simulink model "Roll_Autopilot"  (R2017b)
settings: Solver=VariableStepAuto  StartTime=0.0  StopTime=10.0  RelTol=1e-3
model workspace (MAT data in the model file):
  MCOS : class17 (value not decoded)
undefined symbols (not defined in the file): contractAfterSimulation, contractBeforeSimulation, ContractBlock, ContractEnsureBlock, ContractGuaranteeBlock, ContractModeBlock, ContractRequireBlock, ContractValidatorBlock, saveValidatorParameters, Ts
libraries: cocosimLibs x20, simulink x2
(part 2 of 2)

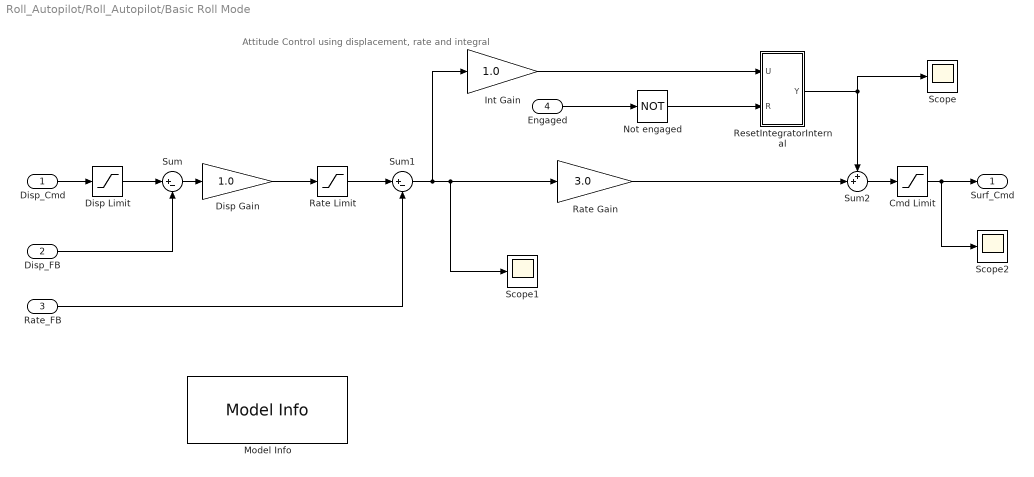
== system Roll_Autopilot/Roll_Autopilot/Basic Roll Mode ==
  note: Attitude Control using displacement, rate and integral
  Disp_Cmd : Inport  OutDataTypeStr=double  PortDimensions=1
  "Disp_FB " : Inport  Port=2  OutDataTypeStr=double  PortDimensions=1  SampleTime=1/40
  Rate_FB : Inport  Port=3  OutDataTypeStr=double  PortDimensions=1  SampleTime=1/40
  Engaged : Inport  Port=4  OutDataTypeStr=boolean  PortDimensions=1  SampleTime=1/40
  Cmd Limit : Saturate  UpperLimit=15  LowerLimit=-15
      settings: AttributesFormatString=%<LowerLimit> to %<UpperLimit> (deg)
  Disp Gain : Gain  Gain=1.0
  Disp Limit : Saturate  UpperLimit=30  LowerLimit=-30
      settings: AttributesFormatString=%<LowerLimit> to %<UpperLimit> (deg)
  Int Gain : Gain  Gain=1.0
  Model Info : simulink/Model-Wide Utilities/Model Info  Frame=on  DisplayStringWithTags=|  HorizontalTextAlignment=Left  LeftAlignmentValue=0.02
      | Attitude Controller
      | Author: %<LastModifiedBy>
      | Version: %<ModelVersion>
      | Date: %<LastModificationDate>
  Not engaged : Logic  Operator=NOT  IconShape=distinctive  AllPortsSameDT=off  OutDataTypeStr=boolean
  Rate Gain : Gain  Gain=3.0
  Rate Limit : Saturate  UpperLimit=6  LowerLimit=-6
      settings: AttributesFormatString=%<LowerLimit> to %<UpperLimit> (deg/sec)
  ResetIntegratorInternal : Subsystem
  Scope : Scope
  Scope1 : Scope
  Scope2 : Scope
  Sum : Sum  Inputs=|+-
  Sum1 : Sum  Inputs=|+-
  Sum2 : Sum  Inputs=++|
  Surf_Cmd : Outport  OutDataTypeStr=double  PortDimensions=1  SampleTime=1/40  VectorParamsAs1DForOutWhenUnconnected=off
  wires:
  Engaged/1 -> Not engaged/1
  Disp_Cmd/1 -> Disp Limit/1
  Rate Limit/1 -> Sum1/1
  ResetIntegratorInternal/1(Y) -> Sum2/1, Scope/1
  Not engaged/1 -> ResetIntegratorInternal/2(R)
  Rate_FB/1 -> Sum1/2
  Sum1/1 -> Int Gain/1, Scope1/1, Rate Gain/1
  Cmd Limit/1 -> Scope2/1, Surf_Cmd/1
  Rate Gain/1 -> Sum2/2
  Disp Gain/1 -> Rate Limit/1
  Sum/1 -> Disp Gain/1
  "Disp_FB "/1 -> Sum/2
  Disp Limit/1 -> Sum/1
  Sum2/1 -> Cmd Limit/1
  Int Gain/1 -> ResetIntegratorInternal/1(U)

== system Roll_Autopilot/Roll_Autopilot/Heading Mode ==
  Psi Ref : Inport  OutDataTypeStr=double  PortDimensions=1  SampleTime=1/40  Interpolate=off
  Psi : Inport  Port=2  OutDataTypeStr=double  PortDimensions=1  SampleTime=1/40  Interpolate=off
  TAS : Inport  Port=3  OutDataTypeStr=double  PortDimensions=1  SampleTime=1/40  Interpolate=off
  Disp Gain : Gain  Gain=0.015
  Model Info : simulink/Model-Wide Utilities/Model Info  Frame=on  DisplayStringWithTags=|  HorizontalTextAlignment=Left  LeftAlignmentValue=0.02
      | Heading Mode
      | Author: %<LastModifiedBy>
      | Version: %<ModelVersion>
      | Date: %<LastModificationDate>
  Product : Product  RndMeth=Zero
  angle diff : Subsystem
  Phi Cmd : Outport  OutDataTypeStr=double  PortDimensions=1  SampleTime=1/40  VectorParamsAs1DForOutWhenUnconnected=off
  wires:
  Psi Ref/1 -> angle diff/1(plus)
  angle diff/1(diff) -> Disp Gain/1  "hdgError"
  TAS/1 -> Product/2
  Disp Gain/1 -> Product/1
  Psi/1 -> angle diff/2(minus)
  Product/1 -> Phi Cmd/1

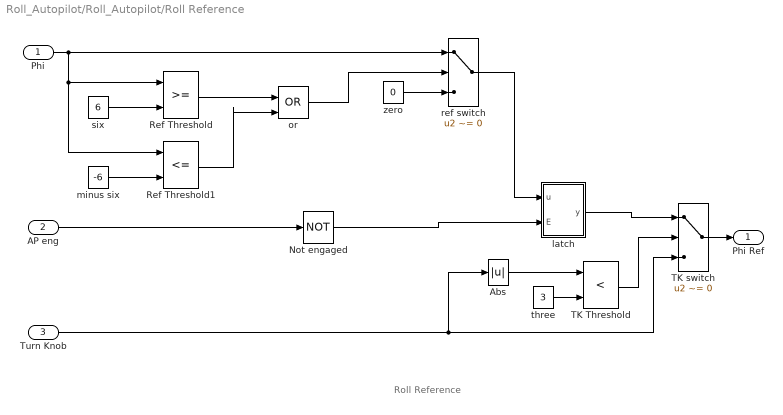
== system Roll_Autopilot/Roll_Autopilot/Roll Reference ==
  note: Roll Reference
  Phi : Inport
  AP eng : Inport  Port=2
  Turn Knob : Inport  Port=3
  Abs : Abs
  Not engaged : Logic  Operator=NOT  IconShape=distinctive  AllPortsSameDT=off  OutDataTypeStr=boolean
  Ref Threshold : RelationalOperator  OutDataTypeStr=boolean  RndMeth=Nearest  InputSameDT=on
  Ref Threshold1 : RelationalOperator  Operator=<=  OutDataTypeStr=boolean  RndMeth=Nearest  InputSameDT=on
  TK Threshold : RelationalOperator  Operator=<  OutDataTypeStr=boolean  RndMeth=Nearest  InputSameDT=on
  TK switch : Switch  Criteria=u2 ~= 0
  latch : Subsystem
  minus six : Constant  Value=-6
  or : Logic  Operator=OR  IconShape=distinctive  OutDataTypeStr=boolean
  ref switch : Switch  Criteria=u2 ~= 0
  six : Constant  Value=6
  three : Constant  Value=3  OutDataTypeStr=double
  zero : Constant  Value=0
  Phi Ref : Outport  VectorParamsAs1DForOutWhenUnconnected=off
  wires:
  minus six/1 -> Ref Threshold1/2
  Ref Threshold1/1 -> or/2
  Ref Threshold/1 -> or/1
  or/1 -> ref switch/2
  zero/1 -> ref switch/3
  six/1 -> Ref Threshold/2
  TK switch/1 -> Phi Ref/1
  AP eng/1 -> Not engaged/1
  Phi/1 -> Ref Threshold1/1, Ref Threshold/1, ref switch/1
  Abs/1 -> TK Threshold/1
  three/1 -> TK Threshold/2
  Turn Knob/1 -> Abs/1, TK switch/3
  TK Threshold/1 -> TK switch/2
  latch/1(y) -> TK switch/1
  ref switch/1 -> latch/1(u)
  Not engaged/1 -> latch/2(E)

== system Roll_Autopilot/Roll_Autopilot_RollAutopilotSpec1/AP-001 ==
  In1 : Inport
  guarantee : Outport  OutDataTypeStr=boolean
  wires:
  In1/1 -> guarantee/1

== system Roll_Autopilot/Roll_Autopilot_RollAutopilotSpec1/AP-003A ==
  In1 : Inport
  guarantee : Outport  OutDataTypeStr=boolean
  wires:
  In1/1 -> guarantee/1

== system Roll_Autopilot/Roll_Autopilot_RollAutopilotSpec1/AP-003B ==
  In1 : Inport
  guarantee : Outport  OutDataTypeStr=boolean
  wires:
  In1/1 -> guarantee/1

== system Roll_Autopilot/Roll_Autopilot_RollAutopilotSpec1/AP-003C ==
  In1 : Inport
  guarantee : Outport  OutDataTypeStr=boolean
  wires:
  In1/1 -> guarantee/1

== system Roll_Autopilot/Roll_Autopilot_RollAutopilotSpec1/AP-003D ==
  In1 : Inport
  guarantee : Outport  OutDataTypeStr=boolean
  wires:
  In1/1 -> guarantee/1

== system Roll_Autopilot/Roll_Autopilot_RollAutopilotSpec1/AP-007 ==
  In1 : Inport
  guarantee : Outport  OutDataTypeStr=boolean
  wires:
  In1/1 -> guarantee/1

== system Roll_Autopilot/Roll_Autopilot_RollAutopilotSpec1/H_call ==
  H_X : Inport  OutDataTypeStr=boolean
  Arrow_xxH_1_ni_23 : Delay  DelayLength=1  InitialCondition=1
  PRE_xxH_2 : Delay  DelayLength=1  InitialCondition=0
  branch_6_IF : Switch  Criteria=u2 ~= 0
  xxH_1_ni_23_init : Constant  Value=0  OutDataTypeStr=boolean
  xxH_3_operator : Logic  AllPortsSameDT=off  OutDataTypeStr=boolean
  H_Y : Outport
  wires:
  PRE_xxH_2/1 -> xxH_3_operator/2
  xxH_3_operator/1 -> branch_6_IF/3
  Arrow_xxH_1_ni_23/1 -> branch_6_IF/2
  xxH_1_ni_23_init/1 -> Arrow_xxH_1_ni_23/1
  branch_6_IF/1 -> H_Y/1, PRE_xxH_2/1
  H_X/1 -> xxH_3_operator/1, branch_6_IF/1

== system Roll_Autopilot/Roll_Autopilot_RollAutopilotSpec1/H_call1 ==
  H_X : Inport  OutDataTypeStr=boolean
  Arrow_xxH_1_ni_23 : Delay  DelayLength=1  InitialCondition=1
  PRE_xxH_2 : Delay  DelayLength=1  InitialCondition=0
  branch_6_IF : Switch  Criteria=u2 ~= 0
  xxH_1_ni_23_init : Constant  Value=0  OutDataTypeStr=boolean
  xxH_3_operator : Logic  AllPortsSameDT=off  OutDataTypeStr=boolean
  H_Y : Outport
  wires:
  PRE_xxH_2/1 -> xxH_3_operator/2
  xxH_3_operator/1 -> branch_6_IF/3
  Arrow_xxH_1_ni_23/1 -> branch_6_IF/2
  xxH_1_ni_23_init/1 -> Arrow_xxH_1_ni_23/1
  branch_6_IF/1 -> H_Y/1, PRE_xxH_2/1
  H_X/1 -> xxH_3_operator/1, branch_6_IF/1

== system Roll_Autopilot/Roll_Autopilot_RollAutopilotSpec1/H_call11 ==
  H_X : Inport  OutDataTypeStr=boolean
  Arrow_xxH_1_ni_23 : Delay  DelayLength=1  InitialCondition=1
  PRE_xxH_2 : Delay  DelayLength=1  InitialCondition=0
  branch_6_IF : Switch  Criteria=u2 ~= 0
  xxH_1_ni_23_init : Constant  Value=0  OutDataTypeStr=boolean
  xxH_3_operator : Logic  AllPortsSameDT=off  OutDataTypeStr=boolean
  H_Y : Outport
  wires:
  PRE_xxH_2/1 -> xxH_3_operator/2
  xxH_3_operator/1 -> branch_6_IF/3
  Arrow_xxH_1_ni_23/1 -> branch_6_IF/2
  xxH_1_ni_23_init/1 -> Arrow_xxH_1_ni_23/1
  branch_6_IF/1 -> H_Y/1, PRE_xxH_2/1
  H_X/1 -> xxH_3_operator/1, branch_6_IF/1

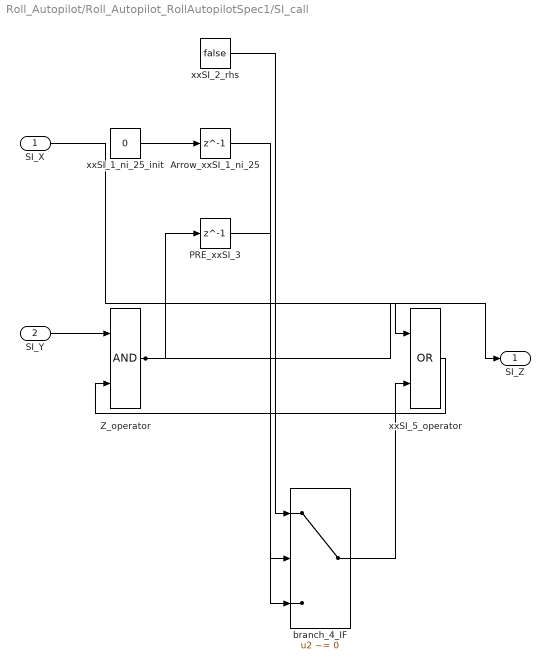
== system Roll_Autopilot/Roll_Autopilot_RollAutopilotSpec1/SI_call ==
  SI_X : Inport  OutDataTypeStr=boolean
  SI_Y : Inport  Port=2  OutDataTypeStr=boolean
  Arrow_xxSI_1_ni_25 : Delay  DelayLength=1  InitialCondition=1
  PRE_xxSI_3 : Delay  DelayLength=1  InitialCondition=0
  Z_operator : Logic  AllPortsSameDT=off  OutDataTypeStr=boolean
  branch_4_IF : Switch  Criteria=u2 ~= 0
  xxSI_1_ni_25_init : Constant  Value=0  OutDataTypeStr=boolean
  xxSI_2_rhs : Constant  Value=false  OutDataTypeStr=boolean
  xxSI_5_operator : Logic  Operator=OR  AllPortsSameDT=off  OutDataTypeStr=boolean
  SI_Z : Outport
  wires:
  branch_4_IF/1 -> xxSI_5_operator/2
  SI_X/1 -> xxSI_5_operator/1
  PRE_xxSI_3/1 -> branch_4_IF/3
  Arrow_xxSI_1_ni_25/1 -> branch_4_IF/2
  xxSI_2_rhs/1 -> branch_4_IF/1
  xxSI_5_operator/1 -> Z_operator/2
  SI_Y/1 -> Z_operator/1
  xxSI_1_ni_25_init/1 -> Arrow_xxSI_1_ni_25/1
  Z_operator/1 -> SI_Z/1, PRE_xxSI_3/1

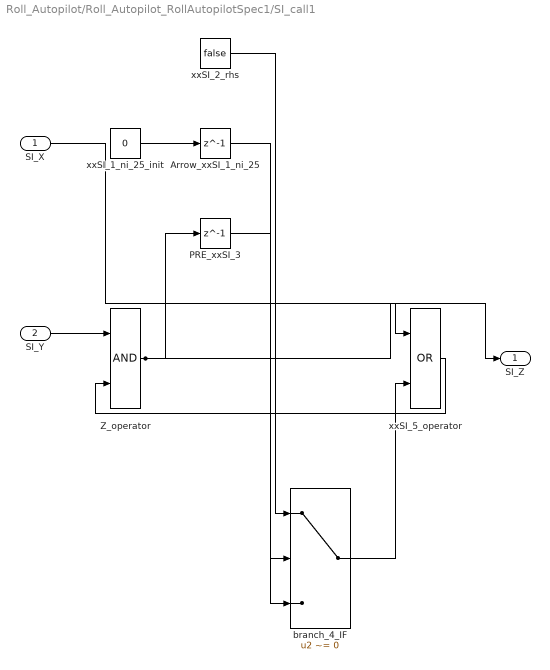
== system Roll_Autopilot/Roll_Autopilot_RollAutopilotSpec1/SI_call1 ==
  SI_X : Inport  OutDataTypeStr=boolean
  SI_Y : Inport  Port=2  OutDataTypeStr=boolean
  Arrow_xxSI_1_ni_25 : Delay  DelayLength=1  InitialCondition=1
  PRE_xxSI_3 : Delay  DelayLength=1  InitialCondition=0
  Z_operator : Logic  AllPortsSameDT=off  OutDataTypeStr=boolean
  branch_4_IF : Switch  Criteria=u2 ~= 0
  xxSI_1_ni_25_init : Constant  Value=0  OutDataTypeStr=boolean
  xxSI_2_rhs : Constant  Value=false  OutDataTypeStr=boolean
  xxSI_5_operator : Logic  Operator=OR  AllPortsSameDT=off  OutDataTypeStr=boolean
  SI_Z : Outport
  wires:
  branch_4_IF/1 -> xxSI_5_operator/2
  SI_X/1 -> xxSI_5_operator/1
  PRE_xxSI_3/1 -> branch_4_IF/3
  Arrow_xxSI_1_ni_25/1 -> branch_4_IF/2
  xxSI_2_rhs/1 -> branch_4_IF/1
  xxSI_5_operator/1 -> Z_operator/2
  SI_Y/1 -> Z_operator/1
  xxSI_1_ni_25_init/1 -> Arrow_xxSI_1_ni_25/1
  Z_operator/1 -> SI_Z/1, PRE_xxSI_3/1

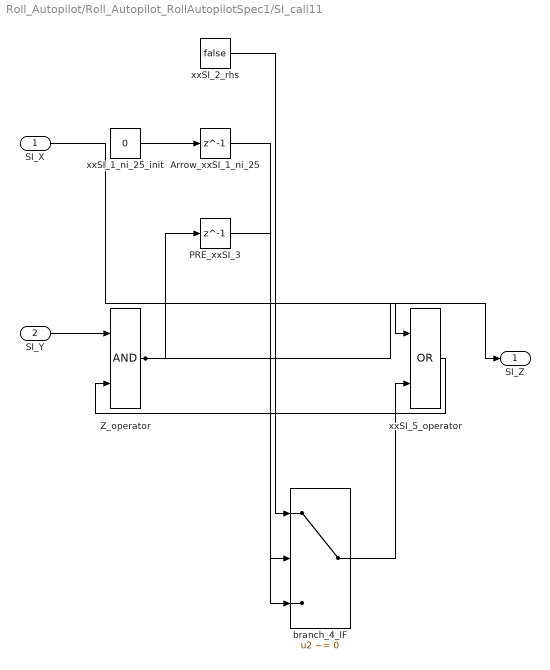
== system Roll_Autopilot/Roll_Autopilot_RollAutopilotSpec1/SI_call11 ==
  SI_X : Inport  OutDataTypeStr=boolean
  SI_Y : Inport  Port=2  OutDataTypeStr=boolean
  Arrow_xxSI_1_ni_25 : Delay  DelayLength=1  InitialCondition=1
  PRE_xxSI_3 : Delay  DelayLength=1  InitialCondition=0
  Z_operator : Logic  AllPortsSameDT=off  OutDataTypeStr=boolean
  branch_4_IF : Switch  Criteria=u2 ~= 0
  xxSI_1_ni_25_init : Constant  Value=0  OutDataTypeStr=boolean
  xxSI_2_rhs : Constant  Value=false  OutDataTypeStr=boolean
  xxSI_5_operator : Logic  Operator=OR  AllPortsSameDT=off  OutDataTypeStr=boolean
  SI_Z : Outport
  wires:
  branch_4_IF/1 -> xxSI_5_operator/2
  SI_X/1 -> xxSI_5_operator/1
  PRE_xxSI_3/1 -> branch_4_IF/3
  Arrow_xxSI_1_ni_25/1 -> branch_4_IF/2
  xxSI_2_rhs/1 -> branch_4_IF/1
  xxSI_5_operator/1 -> Z_operator/2
  SI_Y/1 -> Z_operator/1
  xxSI_1_ni_25_init/1 -> Arrow_xxSI_1_ni_25/1
  Z_operator/1 -> SI_Z/1, PRE_xxSI_3/1

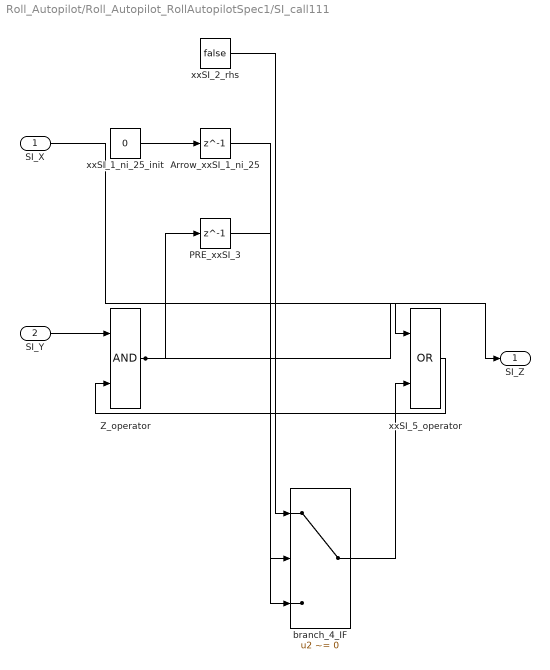
== system Roll_Autopilot/Roll_Autopilot_RollAutopilotSpec1/SI_call111 ==
  SI_X : Inport  OutDataTypeStr=boolean
  SI_Y : Inport  Port=2  OutDataTypeStr=boolean
  Arrow_xxSI_1_ni_25 : Delay  DelayLength=1  InitialCondition=1
  PRE_xxSI_3 : Delay  DelayLength=1  InitialCondition=0
  Z_operator : Logic  AllPortsSameDT=off  OutDataTypeStr=boolean
  branch_4_IF : Switch  Criteria=u2 ~= 0
  xxSI_1_ni_25_init : Constant  Value=0  OutDataTypeStr=boolean
  xxSI_2_rhs : Constant  Value=false  OutDataTypeStr=boolean
  xxSI_5_operator : Logic  Operator=OR  AllPortsSameDT=off  OutDataTypeStr=boolean
  SI_Z : Outport
  wires:
  branch_4_IF/1 -> xxSI_5_operator/2
  SI_X/1 -> xxSI_5_operator/1
  PRE_xxSI_3/1 -> branch_4_IF/3
  Arrow_xxSI_1_ni_25/1 -> branch_4_IF/2
  xxSI_2_rhs/1 -> branch_4_IF/1
  xxSI_5_operator/1 -> Z_operator/2
  SI_Y/1 -> Z_operator/1
  xxSI_1_ni_25_init/1 -> Arrow_xxSI_1_ni_25/1
  Z_operator/1 -> SI_Z/1, PRE_xxSI_3/1

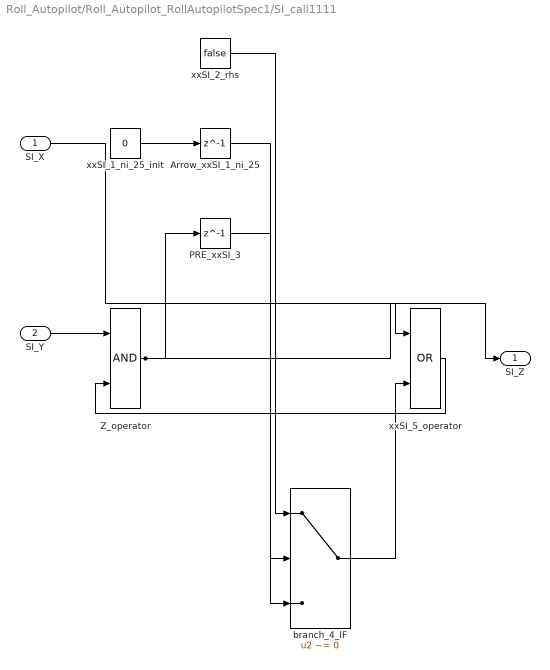
== system Roll_Autopilot/Roll_Autopilot_RollAutopilotSpec1/SI_call1111 ==
  SI_X : Inport  OutDataTypeStr=boolean
  SI_Y : Inport  Port=2  OutDataTypeStr=boolean
  Arrow_xxSI_1_ni_25 : Delay  DelayLength=1  InitialCondition=1
  PRE_xxSI_3 : Delay  DelayLength=1  InitialCondition=0
  Z_operator : Logic  AllPortsSameDT=off  OutDataTypeStr=boolean
  branch_4_IF : Switch  Criteria=u2 ~= 0
  xxSI_1_ni_25_init : Constant  Value=0  OutDataTypeStr=boolean
  xxSI_2_rhs : Constant  Value=false  OutDataTypeStr=boolean
  xxSI_5_operator : Logic  Operator=OR  AllPortsSameDT=off  OutDataTypeStr=boolean
  SI_Z : Outport
  wires:
  branch_4_IF/1 -> xxSI_5_operator/2
  SI_X/1 -> xxSI_5_operator/1
  PRE_xxSI_3/1 -> branch_4_IF/3
  Arrow_xxSI_1_ni_25/1 -> branch_4_IF/2
  xxSI_2_rhs/1 -> branch_4_IF/1
  xxSI_5_operator/1 -> Z_operator/2
  SI_Y/1 -> Z_operator/1
  xxSI_1_ni_25_init/1 -> Arrow_xxSI_1_ni_25/1
  Z_operator/1 -> SI_Z/1, PRE_xxSI_3/1

== system Roll_Autopilot/Roll_Autopilot_RollAutopilotSpec1/SI_call11111 ==
  SI_X : Inport  OutDataTypeStr=boolean
  SI_Y : Inport  Port=2  OutDataTypeStr=boolean
  Arrow_xxSI_1_ni_25 : Delay  DelayLength=1  InitialCondition=1
  PRE_xxSI_3 : Delay  DelayLength=1  InitialCondition=0
  Z_operator : Logic  AllPortsSameDT=off  OutDataTypeStr=boolean
  branch_4_IF : Switch  Criteria=u2 ~= 0
  xxSI_1_ni_25_init : Constant  Value=0  OutDataTypeStr=boolean
  xxSI_2_rhs : Constant  Value=false  OutDataTypeStr=boolean
  xxSI_5_operator : Logic  Operator=OR  AllPortsSameDT=off  OutDataTypeStr=boolean
  SI_Z : Outport
  wires:
  branch_4_IF/1 -> xxSI_5_operator/2
  SI_X/1 -> xxSI_5_operator/1
  PRE_xxSI_3/1 -> branch_4_IF/3
  Arrow_xxSI_1_ni_25/1 -> branch_4_IF/2
  xxSI_2_rhs/1 -> branch_4_IF/1
  xxSI_5_operator/1 -> Z_operator/2
  SI_Y/1 -> Z_operator/1
  xxSI_1_ni_25_init/1 -> Arrow_xxSI_1_ni_25/1
  Z_operator/1 -> SI_Z/1, PRE_xxSI_3/1

== system Roll_Autopilot/Roll_Autopilot_RollAutopilotSpec1/SI_call111111 ==
  SI_X : Inport  OutDataTypeStr=boolean
  SI_Y : Inport  Port=2  OutDataTypeStr=boolean
  Arrow_xxSI_1_ni_25 : Delay  DelayLength=1  InitialCondition=1
  PRE_xxSI_3 : Delay  DelayLength=1  InitialCondition=0
  Z_operator : Logic  AllPortsSameDT=off  OutDataTypeStr=boolean
  branch_4_IF : Switch  Criteria=u2 ~= 0
  xxSI_1_ni_25_init : Constant  Value=0  OutDataTypeStr=boolean
  xxSI_2_rhs : Constant  Value=false  OutDataTypeStr=boolean
  xxSI_5_operator : Logic  Operator=OR  AllPortsSameDT=off  OutDataTypeStr=boolean
  SI_Z : Outport
  wires:
  branch_4_IF/1 -> xxSI_5_operator/2
  SI_X/1 -> xxSI_5_operator/1
  PRE_xxSI_3/1 -> branch_4_IF/3
  Arrow_xxSI_1_ni_25/1 -> branch_4_IF/2
  xxSI_2_rhs/1 -> branch_4_IF/1
  xxSI_5_operator/1 -> Z_operator/2
  SI_Y/1 -> Z_operator/1
  xxSI_1_ni_25_init/1 -> Arrow_xxSI_1_ni_25/1
  Z_operator/1 -> SI_Z/1, PRE_xxSI_3/1

== system Roll_Autopilot/Roll_Autopilot_RollAutopilotSpec1/SI_call1111111 ==
  SI_X : Inport  OutDataTypeStr=boolean
  SI_Y : Inport  Port=2  OutDataTypeStr=boolean
  Arrow_xxSI_1_ni_25 : Delay  DelayLength=1  InitialCondition=1
  PRE_xxSI_3 : Delay  DelayLength=1  InitialCondition=0
  Z_operator : Logic  AllPortsSameDT=off  OutDataTypeStr=boolean
  branch_4_IF : Switch  Criteria=u2 ~= 0
  xxSI_1_ni_25_init : Constant  Value=0  OutDataTypeStr=boolean
  xxSI_2_rhs : Constant  Value=false  OutDataTypeStr=boolean
  xxSI_5_operator : Logic  Operator=OR  AllPortsSameDT=off  OutDataTypeStr=boolean
  SI_Z : Outport
  wires:
  branch_4_IF/1 -> xxSI_5_operator/2
  SI_X/1 -> xxSI_5_operator/1
  PRE_xxSI_3/1 -> branch_4_IF/3
  Arrow_xxSI_1_ni_25/1 -> branch_4_IF/2
  xxSI_2_rhs/1 -> branch_4_IF/1
  xxSI_5_operator/1 -> Z_operator/2
  SI_Y/1 -> Z_operator/1
  xxSI_1_ni_25_init/1 -> Arrow_xxSI_1_ni_25/1
  Z_operator/1 -> SI_Z/1, PRE_xxSI_3/1

== system Roll_Autopilot/Roll_Autopilot_RollAutopilotSpec1/SI_call11111111 ==
  SI_X : Inport  OutDataTypeStr=boolean
  SI_Y : Inport  Port=2  OutDataTypeStr=boolean
  Arrow_xxSI_1_ni_25 : Delay  DelayLength=1  InitialCondition=1
  PRE_xxSI_3 : Delay  DelayLength=1  InitialCondition=0
  Z_operator : Logic  AllPortsSameDT=off  OutDataTypeStr=boolean
  branch_4_IF : Switch  Criteria=u2 ~= 0
  xxSI_1_ni_25_init : Constant  Value=0  OutDataTypeStr=boolean
  xxSI_2_rhs : Constant  Value=false  OutDataTypeStr=boolean
  xxSI_5_operator : Logic  Operator=OR  AllPortsSameDT=off  OutDataTypeStr=boolean
  SI_Z : Outport
  wires:
  branch_4_IF/1 -> xxSI_5_operator/2
  SI_X/1 -> xxSI_5_operator/1
  PRE_xxSI_3/1 -> branch_4_IF/3
  Arrow_xxSI_1_ni_25/1 -> branch_4_IF/2
  xxSI_2_rhs/1 -> branch_4_IF/1
  xxSI_5_operator/1 -> Z_operator/2
  SI_Y/1 -> Z_operator/1
  xxSI_1_ni_25_init/1 -> Arrow_xxSI_1_ni_25/1
  Z_operator/1 -> SI_Z/1, PRE_xxSI_3/1

== system Roll_Autopilot/Roll_Autopilot_RollAutopilotSpec1/hdg_hold_mode ==
  note: Shouldn't not be edited
  require : Inport  OutDataTypeStr=boolean
  ensure : Inport  Port=2  OutDataTypeStr=boolean
  and : Logic  Operator=NOT  IconShape=distinctive  AllPortsSameDT=off  OutDataTypeStr=boolean
  or : Logic  Operator=OR  IconShape=distinctive  AllPortsSameDT=off  OutDataTypeStr=boolean
  mode : Outport
  wires:
  or/1 -> mode/1
  ensure/1 -> or/2
  and/1 -> or/1
  require/1 -> and/1

== system Roll_Autopilot/Roll_Autopilot_RollAutopilotSpec1/hdg_hold_mode_ensure ==
  In1 : Inport
  ensure : Outport  OutDataTypeStr=boolean
  wires:
  In1/1 -> ensure/1

== system Roll_Autopilot/Roll_Autopilot_RollAutopilotSpec1/hdg_hold_mode_require ==
  In1 : Inport
  require : Outport  OutDataTypeStr=boolean
  wires:
  In1/1 -> require/1

== system Roll_Autopilot/Roll_Autopilot_RollAutopilotSpec1/roll_hold_mode ==
  note: Shouldn't not be edited
  require : Inport  OutDataTypeStr=boolean
  ensure : Inport  Port=2  OutDataTypeStr=boolean
  and : Logic  Operator=NOT  IconShape=distinctive  AllPortsSameDT=off  OutDataTypeStr=boolean
  or : Logic  Operator=OR  IconShape=distinctive  AllPortsSameDT=off  OutDataTypeStr=boolean
  mode : Outport
  wires:
  or/1 -> mode/1
  ensure/1 -> or/2
  and/1 -> or/1
  require/1 -> and/1

== system Roll_Autopilot/Roll_Autopilot_RollAutopilotSpec1/roll_hold_mode_ensure ==
  In1 : Inport
  ensure : Outport  OutDataTypeStr=boolean
  wires:
  In1/1 -> ensure/1

== system Roll_Autopilot/Roll_Autopilot_RollAutopilotSpec1/roll_hold_mode_require ==
  In1 : Inport
  require : Outport  OutDataTypeStr=boolean
  wires:
  In1/1 -> require/1

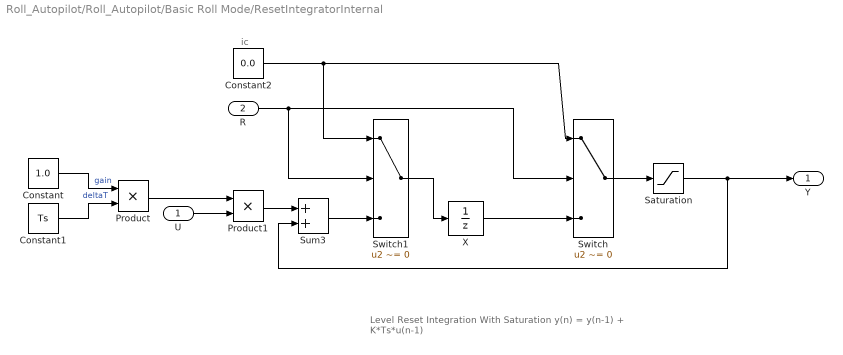
== system Roll_Autopilot/Roll_Autopilot/Basic Roll Mode/ResetIntegratorInternal ==
  note: ic
  note: Level Reset Integration With Saturation
      | y(n) = y(n-1) + K*Ts*u(n-1)
  U : Inport
  R : Inport  Port=2
  Constant : Constant  Value=1.0
  Constant1 : Constant  Value=Ts
  Constant2 : Constant  Value=0.0
  Product : Product  RndMeth=Zero
  Product1 : Product  RndMeth=Zero
  Saturation : Saturate  UpperLimit=5  LowerLimit=-5
  Sum3 : Sum
  Switch : Switch  Criteria=u2 ~= 0
  Switch1 : Switch  Criteria=u2 ~= 0
  X : UnitDelay  SampleTime=Ts  HasFrameUpgradeWarning=on
  Y : Outport  VectorParamsAs1DForOutWhenUnconnected=off
  wires:
  Product1/1 -> Sum3/1
  U/1 -> Product1/2
  Sum3/1 -> Switch1/3
  Product/1 -> Product1/1
  Switch/1 -> Saturation/1
  Constant2/1 -> Switch1/1, Switch/1
  Constant1/1 -> Product/2  "deltaT"
  Switch1/1 -> X/1
  Constant/1 -> Product/1  "gain"
  Saturation/1 -> Y/1, Sum3/2
  R/1 -> Switch1/2, Switch/2
  X/1 -> Switch/3

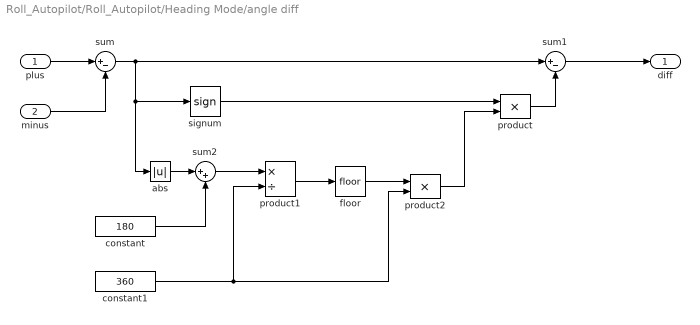
== system Roll_Autopilot/Roll_Autopilot/Heading Mode/angle diff ==
  plus : Inport  OutDataTypeStr=double
  minus : Inport  Port=2  OutDataTypeStr=double
  abs : Abs  ZeroCross=off
  constant : Constant  Value=180
  constant1 : Constant  Value=360
  floor : Rounding
  product : Product  RndMeth=Zero  InputSameDT=on  OutDataTypeStr=Inherit: Same as first input
  product1 : Product  Inputs=*/  RndMeth=Zero  InputSameDT=on  OutDataTypeStr=Inherit: Same as first input
  product2 : Product  RndMeth=Zero  InputSameDT=on  OutDataTypeStr=Inherit: Same as first input
  signum : Signum  ZeroCross=off
  sum : Sum  Inputs=|+-  RndMeth=Zero  InputSameDT=on  OutDataTypeStr=Inherit: Same as first input
  sum1 : Sum  Inputs=|+-  RndMeth=Zero  InputSameDT=on  OutDataTypeStr=Inherit: Same as first input
  sum2 : Sum  Inputs=|++  RndMeth=Zero  InputSameDT=on  OutDataTypeStr=Inherit: Same as first input
  diff : Outport  VectorParamsAs1DForOutWhenUnconnected=off
  wires:
  product2/1 -> product/2
  product/1 -> sum1/2
  sum2/1 -> product1/1
  constant/1 -> sum2/2
  sum1/1 -> diff/1
  signum/1 -> product/1
  floor/1 -> product2/1
  minus/1 -> sum/2
  plus/1 -> sum/1
  product1/1 -> floor/1
  sum/1 -> sum1/1, abs/1, signum/1
  abs/1 -> sum2/1
  constant1/1 -> product2/2, product1/2

== system Roll_Autopilot/Roll_Autopilot/Roll Reference/latch ==
  note: Xold
  note: Enable
  u : Inport
  E : Inport  Port=2
  Enable : Switch  Criteria=u2 ~= 0  OutDataTypeStr=Inherit: Inherit via back propagation  ZeroCross=off
  FixPt Unit Delay1 : UnitDelay  SampleTime=Ts
  y : Outport  VectorParamsAs1DForOutWhenUnconnected=off
  wires:
  FixPt Unit Delay1/1 -> y/1, Enable/3
  Enable/1 -> FixPt Unit Delay1/1  "Xnew"
  E/1 -> Enable/2
  u/1 -> Enable/1
